simulink model "logunit"  (Simulink 7.6)
settings: Solver=FixedStepDiscrete  StartTime=0.0  StopTime=2  FixedStep=1/50e6  RelTol=1e-3
libraries: simulink x30
settings Model: Creator=jordan  LastModifiedBy=jordan
settings DataIOCC: LimitDataPoints=off  SaveOutput=off  SignalLogging=off  DSMLogging=off  SaveTime=off
settings OptimizationCC: BlockReduction=off  ConditionallyExecuteInputs=off  InlineParams=on

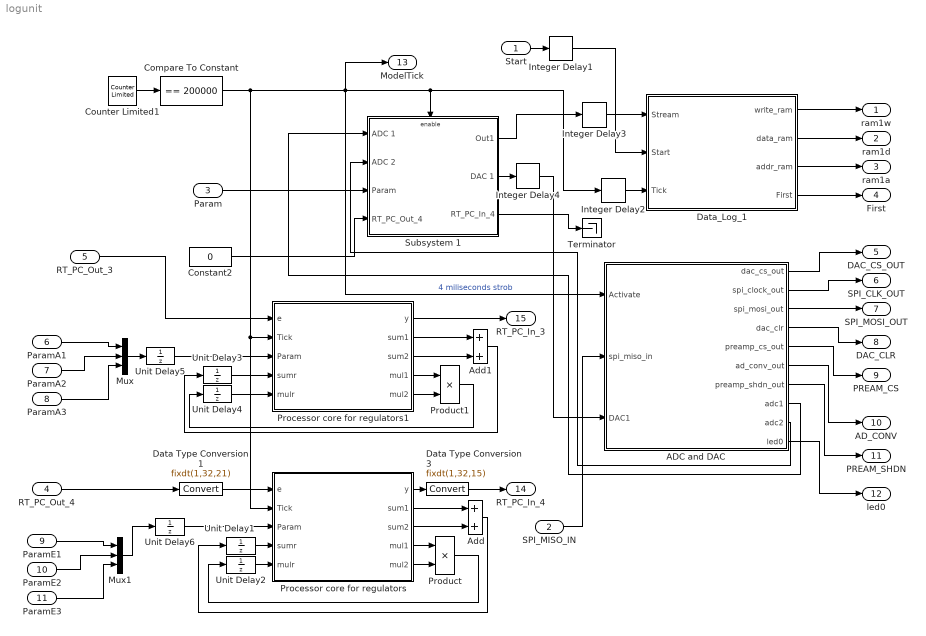
== system logunit ==
  Start : Inport  OutDataTypeStr=boolean
  SPI_MISO_IN : Inport  Port=2  OutDataTypeStr=boolean
  Param : Inport  Port=3  OutDataTypeStr=uint8
  RT_PC_Out_4 : Inport  Port=4  OutDataTypeStr=fixdt(1,32,15)
  RT_PC_Out_3 : Inport  Port=5  OutDataTypeStr=fixdt(1,32,24)
  ParamA1 : Inport  Port=6  OutDataTypeStr=fixdt(1,32,24)  PortDimensions=1
  ParamA2 : Inport  Port=7  OutDataTypeStr=fixdt(1,32,24)  PortDimensions=1
  ParamA3 : Inport  Port=8  OutDataTypeStr=fixdt(1,32,24)  PortDimensions=1
  ParamE1 : Inport  Port=9  OutDataTypeStr=fixdt(1,32,21)  PortDimensions=1
  ParamE2 : Inport  Port=10  OutDataTypeStr=fixdt(1,32,21)  PortDimensions=1
  ParamE3 : Inport  Port=11  OutDataTypeStr=fixdt(1,32,21)  PortDimensions=1
  ADC and DAC : Subsystem
  Add : Sum  AccumDataTypeStr=fixdt(1,32,21)  OutDataTypeStr=fixdt(1,32,21)
  Add1 : Sum  AccumDataTypeStr=fixdt(1,32,24)  OutDataTypeStr=fixdt(1,32,24)
  Compare To Constant : simulink/Logic and Bit Operations/Compare To Constant  SystemSampleTime=-1  relop===  const=200000  LogicOutDataTypeMode=boolean
  Constant2 : Constant  Value=0  OutDataTypeStr=fixdt(1,32,15)
  Counter Limited1 : simulink/Sources/Counter Limited  SystemSampleTime=-1  uplimit=200000  tsamp=-1
  Data Type Conversion1 : DataTypeConversion  OutDataTypeStr=fixdt(1,32,21)
  Data Type Conversion3 : DataTypeConversion  OutDataTypeStr=fixdt(1,32,15)
  Data_Log_1 : Stateflow chart  TreatAsAtomicUnit=on
  Integer Delay{1..4} (4 alike) : simulink/Discrete/Integer Delay  NumDelays=1  vinit=0.0  samptime=-1
  Mux : Mux  Inputs=3
  Mux1 : Mux  Inputs=3
  Processor core for regulators : Stateflow chart  TreatAsAtomicUnit=on
  Processor core for regulators1 : Stateflow chart  TreatAsAtomicUnit=on
  Product : Product  OutDataTypeStr=fixdt(1,32,21)  RndMeth=Zero
  Product1 : Product  OutDataTypeStr=fixdt(1,32,24)  RndMeth=Zero
  Subsystem 1 : Subsystem
  Terminator : Terminator
  Unit Delay{1..6} (6 alike) : UnitDelay  SampleTime=-1
  ram1w : Outport
  ram1d : Outport  Port=2
  ram1a : Outport  Port=3
  First : Outport  Port=4
  DAC_CS_OUT : Outport  Port=5
  SPI_CLK_OUT : Outport  Port=6
  SPI_MOSI_OUT : Outport  Port=7
  DAC_CLR : Outport  Port=8
  PREAM_CS : Outport  Port=9
  AD_CONV : Outport  Port=10
  PREAM_SHDN : Outport  Port=11
  led0 : Outport  Port=12
  ModelTick : Outport  Port=13
  RT_PC_In_4 : Outport  Port=14  OutDataTypeStr=fixdt(1,32,15)
  RT_PC_In_3 : Outport  Port=15  OutDataTypeStr=fixdt(1,32,24)
  wires:
  Start/1 -> Integer Delay1/1
  Data_Log_1/1(write_ram) -> ram1w/1
  Data_Log_1/2(data_ram) -> ram1d/1
  Data_Log_1/3(addr_ram) -> ram1a/1
  Data_Log_1/4(First) -> First/1
  Integer Delay1/1 -> Data_Log_1/2(Start)
  Counter Limited1/1 -> Compare To Constant/1
  Compare To Constant/1 -> Subsystem 1/Enable, Integer Delay2/1, ModelTick/1, ADC and DAC/1(Activate), Processor core for regulators/2(Tick), Processor core for regulators1/2(Tick)  "4 miliseconds strob"
  Integer Delay2/1 -> Data_Log_1/3(Tick)
  Integer Delay3/1 -> Data_Log_1/1(Stream)
  Subsystem 1/1(Out1) -> Integer Delay3/1
  Subsystem 1/2(DAC 1) -> Integer Delay4/1
  SPI_MISO_IN/1 -> ADC and DAC/2(spi_miso_in)
  ADC and DAC/1(dac_cs_out) -> DAC_CS_OUT/1
  ADC and DAC/2(spi_clock_out) -> SPI_CLK_OUT/1
  ADC and DAC/3(spi_mosi_out) -> SPI_MOSI_OUT/1
  ADC and DAC/4(dac_clr) -> DAC_CLR/1
  ADC and DAC/5(preamp_cs_out) -> PREAM_CS/1
  ADC and DAC/6(ad_conv_out) -> AD_CONV/1
  ADC and DAC/7(preamp_shdn_out) -> PREAM_SHDN/1
  ADC and DAC/9(adc2) -> Subsystem 1/2(ADC 2)
  ADC and DAC/8(adc1) -> Subsystem 1/1(ADC 1)
  Integer Delay4/1 -> ADC and DAC/3(DAC1)
  ADC and DAC/10(led0) -> led0/1
  Param/1 -> Subsystem 1/3(Param)
  Constant2/1 -> Subsystem 1/4(RT_PC_Out_4)
  Subsystem 1/3(RT_PC_In_4) -> Terminator/1
  Processor core for regulators/2(sum1) -> Add/1
  Processor core for regulators/4(mul1) -> Product/1
  Processor core for regulators/5(mul2) -> Product/2
  Unit Delay1/1 -> Processor core for regulators/4(sumr)
  Add/1 -> Unit Delay1/1
  Unit Delay6/1 -> Processor core for regulators/3(Param)
  Processor core for regulators/3(sum2) -> Add/2
  Unit Delay2/1 -> Processor core for regulators/5(mulr)
  Product/1 -> Unit Delay2/1
  RT_PC_Out_4/1 -> Data Type Conversion1/1
  Processor core for regulators/1(y) -> Data Type Conversion3/1
  Data Type Conversion3/1 -> RT_PC_In_4/1
  Data Type Conversion1/1 -> Processor core for regulators/1(e)
  RT_PC_Out_3/1 -> Processor core for regulators1/1(e)
  Processor core for regulators1/1(y) -> RT_PC_In_3/1
  Unit Delay5/1 -> Processor core for regulators1/3(Param)
  Processor core for regulators1/2(sum1) -> Add1/1
  Processor core for regulators1/3(sum2) -> Add1/2
  Processor core for regulators1/4(mul1) -> Product1/1
  Processor core for regulators1/5(mul2) -> Product1/2
  Unit Delay3/1 -> Processor core for regulators1/4(sumr)
  Unit Delay4/1 -> Processor core for regulators1/5(mulr)
  Product1/1 -> Unit Delay4/1
  Add1/1 -> Unit Delay3/1
  ParamA1/1 -> Mux/1
  Mux/1 -> Unit Delay5/1
  ParamA2/1 -> Mux/2
  ParamA3/1 -> Mux/3
  ParamE1/1 -> Mux1/1
  ParamE2/1 -> Mux1/2
  ParamE3/1 -> Mux1/3
  Mux1/1 -> Unit Delay6/1

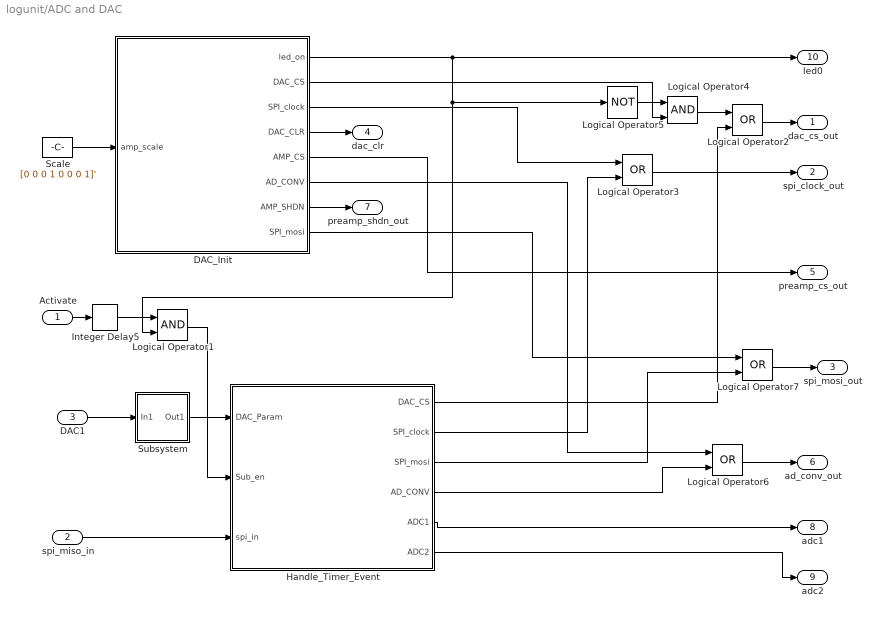
== system logunit/ADC and DAC ==
  Activate : Inport  OutDataTypeStr=boolean
  spi_miso_in : Inport  Port=2  OutDataTypeStr=boolean
  DAC1 : Inport  Port=3  OutDataTypeStr=fixdt(1,12,0)
  DAC_Init : Stateflow chart  TreatAsAtomicUnit=on
  Handle_Timer_Event : Stateflow chart  TreatAsAtomicUnit=on
  Integer Delay5 : simulink/Discrete/Integer Delay  NumDelays=1  vinit=0.0  samptime=-1
  Logical Operator1 : Logic  AllPortsSameDT=off  OutDataTypeStr=boolean
  Logical Operator{2..3,6..7} (4 alike) : Logic  Operator=OR  AllPortsSameDT=off  OutDataTypeStr=boolean
  Logical Operator4 : Logic  AllPortsSameDT=off  OutDataTypeStr=boolean
  Logical Operator5 : Logic  Operator=NOT  AllPortsSameDT=off  OutDataTypeStr=boolean
  Scale : Constant  Value=[0 0 0 1 0 0 0 1]'  OutDataTypeStr=boolean
  Subsystem : Subsystem
  dac_cs_out : Outport
  spi_clock_out : Outport  Port=2
  spi_mosi_out : Outport  Port=3
  dac_clr : Outport  Port=4
  preamp_cs_out : Outport  Port=5
  ad_conv_out : Outport  Port=6
  preamp_shdn_out : Outport  Port=7
  adc1 : Outport  Port=8  OutDataTypeStr=fixdt(1,14,0)
  adc2 : Outport  Port=9  OutDataTypeStr=fixdt(1,14,0)
  led0 : Outport  Port=10
  wires:
  Activate/1 -> Integer Delay5/1
  Subsystem/1(Out1) -> Handle_Timer_Event/1(DAC_Param)
  DAC_Init/1(led_on) -> Logical Operator1/2, Logical Operator5/1, led0/1
  Logical Operator1/1 -> Handle_Timer_Event/2(Sub_en)
  Logical Operator2/1 -> dac_cs_out/1
  DAC_Init/2(DAC_CS) -> Logical Operator4/2
  Logical Operator3/1 -> spi_clock_out/1
  DAC_Init/3(SPI_clock) -> Logical Operator3/1
  Handle_Timer_Event/3(SPI_mosi) -> Logical Operator7/2
  DAC_Init/4(DAC_CLR) -> dac_clr/1
  Logical Operator4/1 -> Logical Operator2/1
  Logical Operator5/1 -> Logical Operator4/1
  DAC_Init/5(AMP_CS) -> preamp_cs_out/1
  DAC_Init/6(AD_CONV) -> Logical Operator6/1
  spi_miso_in/1 -> Handle_Timer_Event/3(spi_in)
  DAC_Init/7(AMP_SHDN) -> preamp_shdn_out/1
  Logical Operator6/1 -> ad_conv_out/1
  Handle_Timer_Event/4(AD_CONV) -> Logical Operator6/2
  Handle_Timer_Event/5(ADC1) -> adc1/1
  Handle_Timer_Event/6(ADC2) -> adc2/1
  DAC1/1 -> Subsystem/1(In1)
  Handle_Timer_Event/1(DAC_CS) -> Logical Operator2/2
  Handle_Timer_Event/2(SPI_clock) -> Logical Operator3/2
  Integer Delay5/1 -> Logical Operator1/1
  Scale/1 -> DAC_Init/1(amp_scale)
  DAC_Init/8(SPI_mosi) -> Logical Operator7/1
  Logical Operator7/1 -> spi_mosi_out/1

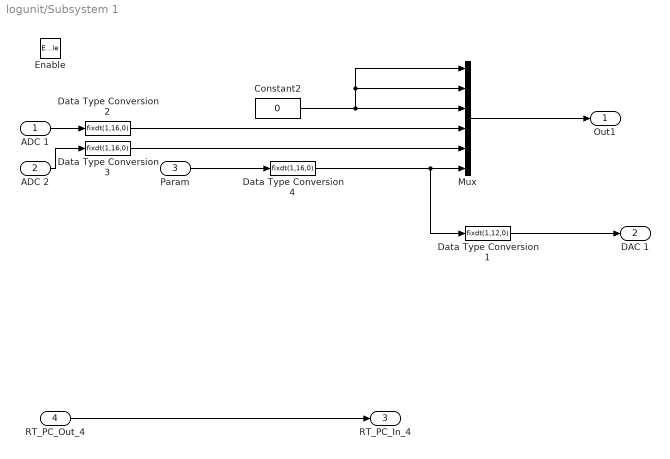
== system logunit/Subsystem 1 ==
  ADC 1 : Inport  OutDataTypeStr=fixdt(1,14,0)
  ADC 2 : Inport  Port=2  OutDataTypeStr=fixdt(1,14,0)
  Param : Inport  Port=3  OutDataTypeStr=uint8
  RT_PC_Out_4 : Inport  Port=4  OutDataTypeStr=fixdt(1,32,15)
  Enable : EnablePort
  Constant2 : Constant  Value=0  OutDataTypeStr=fixdt(1,16,0)
  Data Type Conversion1 : DataTypeConversion  OutDataTypeStr=fixdt(1,12,0)
  Data Type Conversion2 : DataTypeConversion  OutDataTypeStr=fixdt(1,16,0)
  Data Type Conversion3 : DataTypeConversion  OutDataTypeStr=fixdt(1,16,0)
  Data Type Conversion4 : DataTypeConversion  OutDataTypeStr=fixdt(1,16,0)
  Mux : Mux  Inputs=6
  Out1 : Outport  InitialOutput=0
  DAC 1 : Outport  Port=2  OutDataTypeStr=fixdt(1,12,0)  InitialOutput=0
  RT_PC_In_4 : Outport  Port=3  OutDataTypeStr=fixdt(1,32,15)  InitialOutput=0
  wires:
  ADC 1/1 -> Data Type Conversion2/1
  Param/1 -> Data Type Conversion4/1
  Mux/1 -> Out1/1
  ADC 2/1 -> Data Type Conversion3/1
  Data Type Conversion1/1 -> DAC 1/1
  Constant2/1 -> Mux/3, Mux/2, Mux/1
  Data Type Conversion2/1 -> Mux/4
  Data Type Conversion3/1 -> Mux/5
  Data Type Conversion4/1 -> Mux/6, Data Type Conversion1/1
  RT_PC_Out_4/1 -> RT_PC_In_4/1

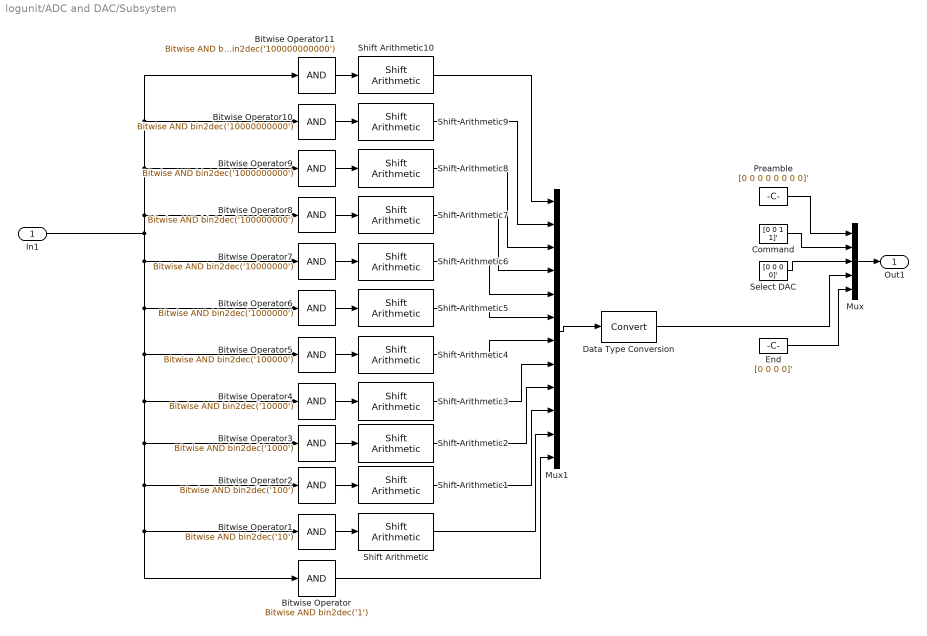
== system logunit/ADC and DAC/Subsystem ==
  In1 : Inport  OutDataTypeStr=fixdt(1,12,0)
  Bitwise Operator : simulink/Logic and Bit Operations/Bitwise Operator  logicop=AND  UseBitMask=on  BitMask=bin2dec('1')  BitMaskRealWorld=Stored Integer
  Bitwise Operator1 : simulink/Logic and Bit Operations/Bitwise Operator  logicop=AND  UseBitMask=on  BitMask=bin2dec('10')  BitMaskRealWorld=Stored Integer
  Bitwise Operator10 : simulink/Logic and Bit Operations/Bitwise Operator  logicop=AND  UseBitMask=on  BitMask=bin2dec('10000000000')  BitMaskRealWorld=Stored Integer
  Bitwise Operator11 : simulink/Logic and Bit Operations/Bitwise Operator  logicop=AND  UseBitMask=on  BitMask=bin2dec('100000000000')  BitMaskRealWorld=Stored Integer
  Bitwise Operator2 : simulink/Logic and Bit Operations/Bitwise Operator  logicop=AND  UseBitMask=on  BitMask=bin2dec('100')  BitMaskRealWorld=Stored Integer
  Bitwise Operator3 : simulink/Logic and Bit Operations/Bitwise Operator  logicop=AND  UseBitMask=on  BitMask=bin2dec('1000')  BitMaskRealWorld=Stored Integer
  Bitwise Operator4 : simulink/Logic and Bit Operations/Bitwise Operator  logicop=AND  UseBitMask=on  BitMask=bin2dec('10000')  BitMaskRealWorld=Stored Integer
  Bitwise Operator5 : simulink/Logic and Bit Operations/Bitwise Operator  logicop=AND  UseBitMask=on  BitMask=bin2dec('100000')  BitMaskRealWorld=Stored Integer
  Bitwise Operator6 : simulink/Logic and Bit Operations/Bitwise Operator  logicop=AND  UseBitMask=on  BitMask=bin2dec('1000000')  BitMaskRealWorld=Stored Integer
  Bitwise Operator7 : simulink/Logic and Bit Operations/Bitwise Operator  logicop=AND  UseBitMask=on  BitMask=bin2dec('10000000')  BitMaskRealWorld=Stored Integer
  Bitwise Operator8 : simulink/Logic and Bit Operations/Bitwise Operator  logicop=AND  UseBitMask=on  BitMask=bin2dec('100000000')  BitMaskRealWorld=Stored Integer
  Bitwise Operator9 : simulink/Logic and Bit Operations/Bitwise Operator  logicop=AND  UseBitMask=on  BitMask=bin2dec('1000000000')  BitMaskRealWorld=Stored Integer
  Command : Constant  Value=[0 0 1 1]'  OutDataTypeStr=boolean
  Data Type Conversion : DataTypeConversion
  End : Constant  Value=[0 0 0 0]'  OutDataTypeStr=boolean
  Mux : Mux  Inputs=5
  Mux1 : Mux  Inputs=12
  Preamble : Constant  Value=[0 0 0 0 0 0 0 0]'  OutDataTypeStr=boolean
  Select DAC : Constant  Value=[0 0 0 0]'  OutDataTypeStr=boolean
  Shift Arithmetic : simulink/Logic and Bit Operations/Shift Arithmetic  SystemSampleTime=-1  nBitShiftRight=1  nBinPtShiftRight=0
  Shift Arithmetic1 : simulink/Logic and Bit Operations/Shift Arithmetic  SystemSampleTime=-1  nBitShiftRight=2  nBinPtShiftRight=0
  Shift Arithmetic10 : simulink/Logic and Bit Operations/Shift Arithmetic  SystemSampleTime=-1  nBitShiftRight=11  nBinPtShiftRight=0
  Shift Arithmetic2 : simulink/Logic and Bit Operations/Shift Arithmetic  SystemSampleTime=-1  nBitShiftRight=3  nBinPtShiftRight=0
  Shift Arithmetic3 : simulink/Logic and Bit Operations/Shift Arithmetic  SystemSampleTime=-1  nBitShiftRight=4  nBinPtShiftRight=0
  Shift Arithmetic4 : simulink/Logic and Bit Operations/Shift Arithmetic  SystemSampleTime=-1  nBitShiftRight=5  nBinPtShiftRight=0
  Shift Arithmetic5 : simulink/Logic and Bit Operations/Shift Arithmetic  SystemSampleTime=-1  nBitShiftRight=6  nBinPtShiftRight=0
  Shift Arithmetic6 : simulink/Logic and Bit Operations/Shift Arithmetic  SystemSampleTime=-1  nBitShiftRight=7  nBinPtShiftRight=0
  Shift Arithmetic7 : simulink/Logic and Bit Operations/Shift Arithmetic  SystemSampleTime=-1  nBitShiftRight=8  nBinPtShiftRight=0
  Shift Arithmetic8 : simulink/Logic and Bit Operations/Shift Arithmetic  SystemSampleTime=-1  nBitShiftRight=9  nBinPtShiftRight=0
  Shift Arithmetic9 : simulink/Logic and Bit Operations/Shift Arithmetic  SystemSampleTime=-1  nBitShiftRight=10  nBinPtShiftRight=0
  Out1 : Outport
  wires:
  Preamble/1 -> Mux/1
  Command/1 -> Mux/2
  Select DAC/1 -> Mux/3
  End/1 -> Mux/5
  Mux/1 -> Out1/1
  In1/1 -> Bitwise Operator11/1, Bitwise Operator10/1, Bitwise Operator9/1, Bitwise Operator8/1, Bitwise Operator7/1, Bitwise Operator6/1, Bitwise Operator5/1, Bitwise Operator4/1, Bitwise Operator3/1, Bitwise Operator2/1, Bitwise Operator/1, Bitwise Operator1/1
  Bitwise Operator1/1 -> Shift Arithmetic/1
  Bitwise Operator2/1 -> Shift Arithmetic1/1
  Bitwise Operator3/1 -> Shift Arithmetic2/1
  Bitwise Operator4/1 -> Shift Arithmetic3/1
  Bitwise Operator5/1 -> Shift Arithmetic4/1
  Bitwise Operator6/1 -> Shift Arithmetic5/1
  Bitwise Operator7/1 -> Shift Arithmetic6/1
  Bitwise Operator8/1 -> Shift Arithmetic7/1
  Bitwise Operator9/1 -> Shift Arithmetic8/1
  Bitwise Operator10/1 -> Shift Arithmetic9/1
  Bitwise Operator11/1 -> Shift Arithmetic10/1
  Bitwise Operator/1 -> Mux1/12
  Shift Arithmetic/1 -> Mux1/11
  Shift Arithmetic1/1 -> Mux1/10
  Shift Arithmetic2/1 -> Mux1/9
  Shift Arithmetic3/1 -> Mux1/8
  Shift Arithmetic4/1 -> Mux1/7
  Shift Arithmetic5/1 -> Mux1/6
  Shift Arithmetic6/1 -> Mux1/5
  Shift Arithmetic7/1 -> Mux1/4
  Shift Arithmetic8/1 -> Mux1/3
  Shift Arithmetic9/1 -> Mux1/2
  Shift Arithmetic10/1 -> Mux1/1
  Mux1/1 -> Data Type Conversion/1
  Data Type Conversion/1 -> Mux/4

== stateflow chart Data_Log_1 ==
  settings: executeAtInitialization=1
  state Wait3
  state Stop
  state Wait2
  state Logging
  state Ready
  state WriteData
  note: Address in ram = First*118+18*Channel+2*Piece+0/1
  (default) -> Stop
  (junction 14) -> (junction 10) [order 1] : [Channel==6]{
      | Piece++;
      | write_ram=0;}
  Logging -> (junction 11) [order 1] : [Tick==1]{Channel=0;}
  Wait2 -> Wait3 : {addr_ram++;
      | data_ram=Stream[Channel]>>8;
      | write_ram=1;}
  WriteData -> Wait2 : {data_ram=Stream[Channel];
      | write_ram=1;}
  Logging -> Ready [order 2] : [Start==0]{addr_ram=0;
      | write_ram=0;}
  Stop -> Logging : [Start==1]{
      | First=0;Channel=0;Piece=0;
      | addr_ram=0;}
  (junction 14) -> (junction 11) [order 2]
  Ready -> Stop : [Start==0]
  (junction 12) -> (junction 13) [order 1] : [First==100]{
      | First=0;
      | Piece=0;}
  (junction 11) -> WriteData : {addr_ram=First*118+18*Channel+2*Piece;}
  (junction 10) -> (junction 12) [order 1] : [Piece==9]{
      | Piece=0;
      | First++}
  (junction 10) -> (junction 12) [order 2]
  Wait3 -> (junction 14) : {Channel++;}
  (junction 13) -> Logging
  (junction 12) -> (junction 13) [order 2]
  data: Stream input fixdt(1,16,0) size=6; write_ram output boolean =0; data_ram output uint8; Start input boolean; addr_ram output fixdt(0,14,0) =0; Channel local fixdt(0,3,0) =0; Tick input boolean; Piece local fixdt(0,4,0); First output uint8

== stateflow chart ADC and DAC/DAC_Init ==
  settings: executeAtInitialization=1
  state DAC_init
  state Led_is_Off
  state Wait6
  state Wait3
  state Wait7
  state Wait8
  state Wait9
  state AMP_Init
  state AMP_Init1
  state Wait1
  state Wait10
  state Wait11
  state Wait12
  state Wait13
  state End_Init
  (default) -> Led_is_Off
  Led_is_Off -> DAC_init : [led_on==0]{SPI_clock=0;
      | DAC_CS=1;
      | DAC_CLR=1;
      | AMP_CS=1; AMP_SHDN=0;/*AMP_SHDN=1;*/
      | AD_CONV=0;
      | ind1=0;}
  Wait6 -> AMP_Init : {DAC_CLR=1;
      | /*led_on=1;*/}
  Wait7 -> (junction 57)
  (junction 58) -> Wait3 : {ind1++;}
  (junction 57) -> (junction 58) [order 1] : [ind1<255]
  (junction 57) -> Wait6 [order 2] : {DAC_CLR=0;}
  DAC_init -> (junction 57)
  Wait3 -> Wait9
  Wait9 -> Wait8
  Wait8 -> Wait7
  End_Init -> Led_is_Off
  AMP_Init -> AMP_Init1 : {ind1=0;
      | AMP_CS=0;
      | SPI_mosi=amp_scale[0];}
  AMP_Init1 -> Wait1
  Wait1 -> Wait10
  Wait10 -> Wait11 : {SPI_clock=1;
      | ind1++;}
  Wait11 -> Wait12
  Wait12 -> Wait13
  (junction 59) -> AMP_Init1 [order 1] : [ind1<8]{
      | SPI_mosi=amp_scale[ind1];}
  Wait13 -> (junction 59) : {SPI_clock=0;}
  (junction 59) -> End_Init [order 2] : {AMP_CS=1;
      | SPI_mosi=0;
      | led_on=1;}
  data: led_on output boolean; DAC_CS output boolean =1; SPI_clock output boolean =0; DAC_CLR output boolean =1; ind1 local uint8; AMP_CS output boolean; AD_CONV output boolean; AMP_SHDN output boolean; amp_scale input boolean size=8; SPI_mosi output boolean

== stateflow chart ADC and DAC/Handle_Timer_Event ==
  settings: executeAtInitialization=1
  state Led_is_On
  state Led_is_Off
  state Wait11
  state Wait1
  state Wait3
  state Wait7
  state Wait12
  state AD_Start
  state Wait9
  state Wait10
  (default) -> Led_is_Off
  Led_is_Off -> Led_is_On : [Sub_en==1]{
      | DAC_CS=0;
      | ind1=0;}
  Wait1 -> Wait7 : {SPI_clock=1;}
  Wait3 -> (junction 103)
  Wait7 -> Wait3 : {ind1++;
      | SPI_clock=0;}
  (junction 103) -> (junction 104) [order 1] : [ind1<32]
  (junction 104) -> Wait1 : {SPI_mosi=DAC_Param[ind1];}
  Led_is_On -> (junction 103)
  (junction 103) -> AD_Start [order 2] : {DAC_CS=1;}
  Wait12 -> Led_is_Off [order 2] : {ADC1=adc_data1;
      | ADC2=adc_data2;}
  (junction 105) -> (junction 106) [order 1] : [(ind1>17)&&(ind1<32)]{
      | adc_data2=adc_data2<<1;
      | adc_data2=adc_data2|spi_in;}
  AD_Start -> Wait9 : {AD_CONV=1;}
  Wait9 -> Wait10 : {AD_CONV=0;
      | adc_data1=0;
      | adc_data2=0;
      | ind1=0;}
  Wait10 -> Wait11 : {SPI_clock=1;}
  Wait11 -> Wait12 : {SPI_clock=0;
      | ind1++;}
  Wait12 -> (junction 105) [order 1] : [ind1<34]
  (junction 105) -> (junction 106) [order 2] : [(ind1>1)&&(ind1<16)]{
      | adc_data1=adc_data1<<1;
      | adc_data1=adc_data1|spi_in;}
  (junction 105) -> (junction 106) [order 3]
  (junction 106) -> Wait10
  data: DAC_CS output boolean =1; SPI_clock output boolean =0; SPI_mosi output boolean; DAC_Param input boolean size=32; ind1 local uint8; Sub_en input boolean; adc_data1 local fixdt(1,14,0); adc_data2 local fixdt(1,14,0); spi_in input boolean; AD_CONV output boolean; ADC1 output fixdt(1,14,0); ADC2 output fixdt(1,14,0)

== stateflow chart Processor core for regulators ==
  settings: executeAtInitialization=1
  state Ready
  state Process
  state Wait
  (default) -> Wait
  Ready -> (junction 143) : {Step++;}
  (junction 143) -> (junction 144) [order 2]
  (junction 143) -> (junction 145) [order 1] : [Step==1]
      | {mul1=Param[0];/*Kp*/
      | mul2=e;}
  (junction 155) -> Wait : {y=sumr;
      | e1=e;ui1=ui;
      | Step=0;}
  (junction 144) -> (junction 146) [order 1] : [Step==2]
      | {up=mulr;
      | mul1=Param[1];/*Ki*/
      | mul2=e1;}
  (junction 144) -> (junction 147) [order 2]
  Process -> Ready
  (junction 147) -> (junction 148) [order 1] : [Step==3]
      | {sum2=mulr;
      | sum1=ui1;}
  (junction 145) -> Process
  (junction 148) -> (junction 146)
  (junction 146) -> (junction 145)
  (junction 147) -> (junction 151) [order 2]
  (junction 151) -> (junction 152) [order 1] : [Step==4]
      | {ui=sumr;
      | sum1=e;sum2=-e1;}
  (junction 152) -> (junction 148)
  (junction 151) -> (junction 149) [order 2]
  (junction 149) -> (junction 150) [order 1] : [Step==5]
      | {mul1=sumr;mul2=Param[2];/*Kd*/;
      | sum1=up;sum2=ui;}
  (junction 150) -> (junction 152)
  Wait -> Ready : [Tick==1]
  (junction 153) -> (junction 154) [order 1] : [Step==6]
      | {sum1=mulr;
      | sum2=sumr;}
  (junction 149) -> (junction 153) [order 2]
  (junction 154) -> (junction 150)
  (junction 153) -> (junction 155) [order 2]
  data: e input fixdt(1,32,21); y output fixdt(1,32,21); Step local uint8 =0; sum1 output fixdt(1,32,21); sum2 output fixdt(1,32,21); mul1 output fixdt(1,32,21); mul2 output fixdt(1,32,21); ui1 local fixdt(1,32,21); e1 local fixdt(1,32,21); Tick input boolean; Param input fixdt(1,32,21) size=3; sumr input fixdt(1,32,21); up local fixdt(1,32,21); ui local fixdt(1,32,21); mulr input fixdt(1,32,21)

== stateflow chart Processor core for regulators1 ==
  settings: executeAtInitialization=1
  state Ready
  state Process
  state Wait
  (default) -> Wait
  Ready -> (junction 199) : {Step++;}
  (junction 199) -> (junction 200) [order 2]
  (junction 199) -> (junction 201) [order 1] : [Step==1]
      | {mul1=Param[0];/*Kp*/
      | mul2=e;}
  (junction 211) -> Wait : {y=sumr;
      | e1=e;ui1=ui;
      | Step=0;}
  (junction 200) -> (junction 202) [order 1] : [Step==2]
      | {up=mulr;
      | mul1=Param[1];/*Ki*/
      | mul2=e1;}
  (junction 200) -> (junction 203) [order 2]
  Process -> Ready
  (junction 203) -> (junction 204) [order 1] : [Step==3]
      | {sum2=mulr;
      | sum1=ui1;}
  (junction 201) -> Process
  (junction 204) -> (junction 202)
  (junction 202) -> (junction 201)
  (junction 203) -> (junction 207) [order 2]
  (junction 207) -> (junction 208) [order 1] : [Step==4]
      | {ui=sumr;
      | sum1=e;sum2=-e1;}
  (junction 208) -> (junction 204)
  (junction 207) -> (junction 205) [order 2]
  (junction 205) -> (junction 206) [order 1] : [Step==5]
      | {mul1=sumr;mul2=Param[2];/*Kd*/;
      | sum1=up;sum2=ui;}
  (junction 206) -> (junction 208)
  Wait -> Ready : [Tick==1]
  (junction 209) -> (junction 210) [order 1] : [Step==6]
      | {sum1=mulr;
      | sum2=sumr;}
  (junction 205) -> (junction 209) [order 2]
  (junction 210) -> (junction 206)
  (junction 209) -> (junction 211) [order 2]
  data: e input fixdt(1,32,24); y output fixdt(1,32,24); Step local uint8 =0; sum1 output fixdt(1,32,24); sum2 output fixdt(1,32,24); mul1 output fixdt(1,32,24); mul2 output fixdt(1,32,24); ui1 local fixdt(1,32,24); e1 local fixdt(1,32,24); Tick input boolean; Param input fixdt(1,32,24) size=3; sumr input fixdt(1,32,24); up local fixdt(1,32,24); ui local fixdt(1,32,24); mulr input fixdt(1,32,24)
